simulink model "accumulator_thermal_model"  (R2021a)
settings: Solver=VariableStepAuto  StartTime=0.0  StopTime=Tend  RelTol=1e-7  AbsTol=1e-7
values from neighbouring files (symbols this model uses):
  AH = 13.5    [HT07_Simulink_Setup.m]    (also in Simulink_Setup.m = 17)
  cellInternalResis = .0018    (= 0.0018)    [Simulink_Setup.m]
  SOC0 = 1    [HT07_Simulink_Setup.m]    (also in Simulink_Setup.m)
  startTempC = 26    [HT07_Simulink_Setup.m]    (also in Simulink_Setup.m = 23.3)
  tabResis = 0.00010*nCell    (= 0.0126)    [HT07_Simulink_Setup.m]    (also in Simulink_Setup.m = 9e-05)
undefined symbols (not defined in the file or in its folder): DiscIntNeverNeededParam, emCurrent
libraries: fl_lib x42, nesl_utility x14, ee_lib x2
settings Model: OrderedModelArguments=off  Creator=elrii  LastModifiedBy=erc
settings SolverCC: AutoScaleAbsTol=off  AlgebraicLoopSolver=TrustRegion
settings DataIOCC: ReturnWorkspaceOutputsName=tp141c3138_a421_409b_bff7_0e00beb78378
settings DebuggingCC: SymbolicDimsDataTypeCodeGenerationDiagnostic=none  SFMachineParentedDataDiag=warning
settings SFSimCC: CustomCodeUndefinedFunction=UseInterfaceOnly
settings SimscapeCC: SimscapeLogType=all  SimscapeLogSimulationStatistics=on  SimscapeLogDataHistory=10000

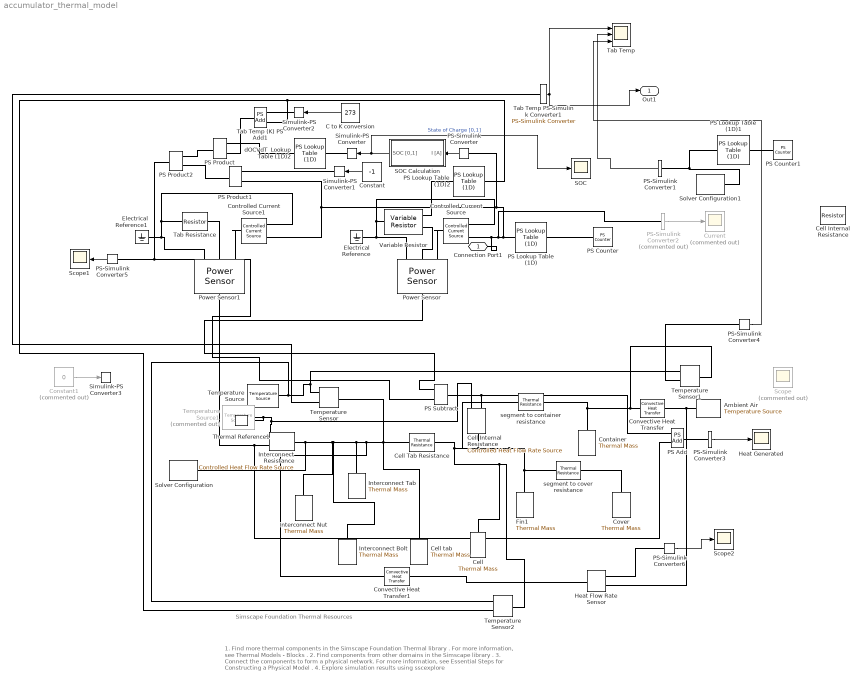
== system accumulator_thermal_model ==
  note: 1. Find more thermal components in the Simscape Foundation Thermal library .
      | For more information, see Thermal Models - Blocks .
      | 2. Find components from other domains in the Simscape library .
      | 3. Connect the components to form a physical network.
      | For more information, see Essential Steps for Constructing a Physical Model .
      | 4. Explore simulation results using sscexplore
  note: Simscape Foundation Thermal Resources
  " Fin1" : fl_lib/Thermal/Thermal Elements/Thermal Mass  mass=mFin kg  sp_heat=cAl J/kg/K  T_specify=on  T_priority=High  T=startTempC degC  T_nominal_specify=off  T_nominal_unit=K  T_nominal_value=1  Q_specify=off  Q_priority=None  Q=0 W  Q_nominal_specify=off  Q_nominal_unit=W  Q_nominal_value=1
  Ambient Air : fl_lib/Thermal/Thermal Sources/Temperature Source  temperature=startTempC degC
  C to K conversion : Constant  Value=273
  "Cell " : fl_lib/Thermal/Thermal Elements/Thermal Mass  mass=mCell kg  sp_heat=cCell J/kg/K  T_specify=on  T_priority=High  T=startTempC degC  T_nominal_specify=off  T_nominal_unit=K  T_nominal_value=1  Q_specify=off  Q_priority=None  Q=0 W  Q_nominal_specify=off  Q_nominal_unit=W  Q_nominal_value=1
  Cell Internal Resistance : fl_lib/Thermal/Thermal Sources/Controlled Heat Flow Rate Source
  "Cell Internal Resistance " : fl_lib/Electrical/Electrical Elements/Resistor  R=cellInternalResis Ohm  i_specify=off  i_priority=None  i=0 A  i_nominal_specify=off  i_nominal_unit=A  i_nominal_value=1  v_specify=off  v_priority=None  v=0 V  v_nominal_specify=off  v_nominal_unit=V  v_nominal_value=1  mask(Resistor){}
  Cell Tab Resistance : fl_lib/Thermal/Thermal Elements/Thermal Resistance  resistance=R_tc K/W  T_specify=off  T_priority=None  T=0 K  T_nominal_specify=off  T_nominal_unit=K  T_nominal_value=1  Q_specify=off  Q_priority=None  Q=0 W  Q_nominal_specify=off  Q_nominal_unit=W  Q_nominal_value=1
      settings: SourceProductBaseCode=SS
  Cell tab : fl_lib/Thermal/Thermal Elements/Thermal Mass  mass=cellTabThermalMass kg  sp_heat=cCu J/kg/K  T_specify=on  T_priority=High  T=startTempC degC  T_nominal_specify=off  T_nominal_unit=K  T_nominal_value=1  Q_specify=off  Q_priority=None  Q=0 W  Q_nominal_specify=off  Q_nominal_unit=W  Q_nominal_value=1
  Constant : Constant  Value=-1
  Constant1 : Constant  Commented=on  Value=0
  Container : fl_lib/Thermal/Thermal Elements/Thermal Mass  mass=mContainerAdj kg  sp_heat=cAl J/kg/K  T_specify=on  T_priority=High  T=startTempC degC  T_nominal_specify=off  T_nominal_unit=K  T_nominal_value=1  Q_specify=off  Q_priority=None  Q=0 W  Q_nominal_specify=off  Q_nominal_unit=W  Q_nominal_value=1
  Controlled Current Source : fl_lib/Electrical/Electrical Sources/Controlled Current Source
  Controlled Current Source1 : fl_lib/Electrical/Electrical Sources/Controlled Current Source
  Convective Heat Transfer : fl_lib/Thermal/Thermal Elements/Convective Heat Transfer  area=convectionArea m^2  heat_tr_coeff=10 W/(m^2 * K)  T_specify=off  T_priority=None  T=0 K  T_nominal_specify=off  T_nominal_unit=K  T_nominal_value=1  Q_specify=off  Q_priority=None  Q=0 W  Q_nominal_specify=off  Q_nominal_unit=W  Q_nominal_value=1
  Convective Heat Transfer1 : fl_lib/Thermal/Thermal Elements/Convective Heat Transfer  area=2.62e-4 m^2  heat_tr_coeff=.001 W/(m^2 * K)  T_specify=off  T_priority=None  T=0 K  T_nominal_specify=off  T_nominal_unit=K  T_nominal_value=1  Q_specify=off  Q_priority=None  Q=0 W  Q_nominal_specify=off  Q_nominal_unit=W  Q_nominal_value=1
  Cover : fl_lib/Thermal/Thermal Elements/Thermal Mass  mass=mCoverAdj kg  sp_heat=cAl J/kg/K  T_specify=on  T_priority=High  T=startTempC degC  T_nominal_specify=off  T_nominal_unit=K  T_nominal_value=1  Q_specify=off  Q_priority=None  Q=0 W  Q_nominal_specify=off  Q_nominal_unit=W  Q_nominal_value=1
  Current : Scope  Commented=on
  Electrical Reference : fl_lib/Electrical/Electrical Elements/Electrical Reference
  Electrical Reference1 : fl_lib/Electrical/Electrical Elements/Electrical Reference
  Heat Flow Rate Sensor : fl_lib/Thermal/Thermal Sensors/Heat Flow Rate Sensor
      settings: SourceProductBaseCode=SS
  Heat Generated : Scope
  Interconnect Bolt : fl_lib/Thermal/Thermal Elements/Thermal Mass  mass=mInterconnectBoltTotal kg  sp_heat=cSt J/kg/K  T_specify=on  T_priority=High  T=startTempC degC  T_nominal_specify=off  T_nominal_unit=K  T_nominal_value=1  Q_specify=off  Q_priority=None  Q=0 W  Q_nominal_specify=off  Q_nominal_unit=W  Q_nominal_value=1
  Interconnect Nut : fl_lib/Thermal/Thermal Elements/Thermal Mass  mass=mInterconnectNutTotal kg  sp_heat=cSt J/kg/K  T_specify=on  T_priority=High  T=startTempC degC  T_nominal_specify=off  T_nominal_unit=K  T_nominal_value=1  Q_specify=off  Q_priority=None  Q=0 W  Q_nominal_specify=off  Q_nominal_unit=W  Q_nominal_value=1
  Interconnect Resistance : fl_lib/Thermal/Thermal Sources/Controlled Heat Flow Rate Source
  Interconnect Tab : fl_lib/Thermal/Thermal Elements/Thermal Mass  mass=mInterconnect kg  sp_heat=cAl J/kg/K  T_specify=on  T_priority=High  T=startTempC degC  T_nominal_specify=off  T_nominal_unit=K  T_nominal_value=1  Q_specify=off  Q_priority=None  Q=0 W  Q_nominal_specify=off  Q_nominal_unit=W  Q_nominal_value=1
  PS Add : fl_lib/Physical Signals/Functions/PS Add
  PS Counter : fl_lib/Physical Signals/Sources/PS Counter  sample_time=1 s  init_val=1  reset_val=0  max_val=100000
      settings: SourceProductBaseCode=SS  InternalSimscapePortConfiguration="{\"Bottom\":[],\"Left\":[],\"Right\":[{\"id\":\"Y\",\"label\":\"Y\",\"type\":\"output\"}],\"Top\":[]}"
  PS Counter1 : fl_lib/Physical Signals/Sources/PS Counter  sample_time=1 s  init_val=1  reset_val=0  max_val=100000
      settings: SourceProductBaseCode=SS  InternalSimscapePortConfiguration="{\"Bottom\":[],\"Left\":[],\"Right\":[{\"id\":\"Y\",\"label\":\"Y\",\"type\":\"output\"}],\"Top\":[]}"
  PS Lookup Table (1D) : fl_lib/Physical Signals/Lookup Tables/PS Lookup Table (1D)  x=emTime  f=-emCurrent A  interp_method=simscape.enum.interpolation.linear  extrap_method=simscape.enum.extrapolation.nearest
      settings: SourceProductBaseCode=SS
  PS Lookup Table (1D)1 : fl_lib/Physical Signals/Lookup Tables/PS Lookup Table (1D)  x=time  f=tempInterp  interp_method=simscape.enum.interpolation.linear  extrap_method=simscape.enum.extrapolation.nearest
      settings: SourceProductBaseCode=SS
  PS Lookup Table (1D)2 : fl_lib/Physical Signals/Lookup Tables/PS Lookup Table (1D)  x=tempVec K  f=IRVec Ohm  interp_method=simscape.enum.interpolation.linear  extrap_method=simscape.enum.extrapolation.linear
      settings: SourceProductBaseCode=SS
  PS Product : fl_lib/Physical Signals/Functions/PS Product
  PS Product1 : fl_lib/Physical Signals/Functions/PS Product
  PS Product2 : fl_lib/Physical Signals/Functions/PS Product
  PS Subtract : fl_lib/Physical Signals/Functions/PS Subtract
  PS-Simulink Converter{,1,3..6} (6 alike) : nesl_utility/PS-Simulink Converter  PhysicalDomain=network_engine_domain  SubClassName=ps_output  LeftPortType=input  RightPortType=output  PseudoPeriodic=off  Frequencies=[]  Unit=inherit  AffineConversion=off
      settings: SourceProductBaseCode=PW,SS
  PS-Simulink Converter2 : nesl_utility/PS-Simulink Converter  Commented=on  PhysicalDomain=network_engine_domain  SubClassName=ps_output  LeftPortType=input  RightPortType=output  PseudoPeriodic=off  Frequencies=[]  Unit=inherit  AffineConversion=off
      settings: SourceProductBaseCode=PW,SS
  Power Sensor : ee_lib/Sensors & Transducers/Power Sensor  measurement_type=1  averaging_period=1e-4 s
      settings: SourceProductBaseCode=PS
  Power Sensor1 : ee_lib/Sensors & Transducers/Power Sensor  measurement_type=1  averaging_period=1e-4 s
      settings: SourceProductBaseCode=PS
  SOC : Scope
  SOC Calculation : Subsystem
  Scope : Scope  Commented=on
  Scope1 : Scope
  Scope2 : Scope
  Simulink-PS Converter : nesl_utility/Simulink-PS Converter  PhysicalDomain=network_engine_domain  SubClassName=ps_input  LeftPortType=input  RightPortType=output  PseudoPeriodic=off  Frequencies=[]  NoiseDistribution=none  NoiseParameters=[]  Unit=1  AffineConversion=off  FilteringAndDerivatives=provide  SimscapeFilterOrder=1  InputFilterTimeConstant=0.001  UdotUserProvided=0
      settings: SourceProductBaseCode=PW,SS
  Simulink-PS Converter1 : nesl_utility/Simulink-PS Converter  PhysicalDomain=network_engine_domain  SubClassName=ps_input  LeftPortType=input  RightPortType=output  PseudoPeriodic=off  Frequencies=[]  NoiseDistribution=none  NoiseParameters=[]  Unit=1  AffineConversion=off  FilteringAndDerivatives=provide  SimscapeFilterOrder=1  InputFilterTimeConstant=0.001  UdotUserProvided=0
      settings: SourceProductBaseCode=PW,SS
  Simulink-PS Converter2 : nesl_utility/Simulink-PS Converter  PhysicalDomain=network_engine_domain  SubClassName=ps_input  LeftPortType=input  RightPortType=output  PseudoPeriodic=off  Frequencies=[]  NoiseDistribution=none  NoiseParameters=[]  Unit=K  AffineConversion=off  FilteringAndDerivatives=provide  SimscapeFilterOrder=1  InputFilterTimeConstant=0.001  UdotUserProvided=0
      settings: SourceProductBaseCode=PW,SS
  Simulink-PS Converter3 : nesl_utility/Simulink-PS Converter  PhysicalDomain=network_engine_domain  SubClassName=ps_input  LeftPortType=input  RightPortType=output  PseudoPeriodic=off  Frequencies=[]  NoiseDistribution=none  NoiseParameters=[]  Unit=W  AffineConversion=off  FilteringAndDerivatives=provide  SimscapeFilterOrder=1  InputFilterTimeConstant=0.001  UdotUserProvided=0
      settings: SourceProductBaseCode=PW,SS
  Solver Configuration : nesl_utility/Solver Configuration  PhysicalDomain=network_engine_domain  SubClassName=solver  LeftPortType=input  RightPortType=generic  Tones=[]  Harmonics=[]  SimulateNoise=off  Profile=off  UseLocalSampling=off  EnableSwitchedLinearOptims=on  FrequencyDomain=off  UseCCode=off  RelTol=0.001  AbsTol=1e-06  MinStep=1e-09  ToWorkspace=off  RevertToSquareIcSolve=off  NumHomotopyIterations=100  PhasorMode=off  PhasorModeNumHarmonics=1  DoDC=off  ResidualTolerance=1e-012  UseLocalSolver=off  LocalSolverChoice=NE_BACKWARD_EULER_ADVANCER  LocalSolverSampleTime=0.001  DoFixedCost=off  MaxNonlinIter=3  MaxModeIter=2  ComputeImpulses=off  ImpulseIterations=2  LinearAlgebra=auto  EquationFormulation=NE_TIME_EF  DelaysMemoryBudget=1024  AutomaticFiltering=on  FilteringTimeConstant=0.001  PartitionStorageMethod=AS_NEEDED  PartitionMemoryBudget=1024  PartitionMethod=ROBUST
      settings: SourceProductBaseCode=PW,SS
  Solver Configuration1 : nesl_utility/Solver Configuration  PhysicalDomain=network_engine_domain  SubClassName=solver  LeftPortType=input  RightPortType=generic  Tones=[]  Harmonics=[]  SimulateNoise=off  Profile=off  UseLocalSampling=off  EnableSwitchedLinearOptims=on  FrequencyDomain=off  UseCCode=off  RelTol=0.001  AbsTol=1e-06  MinStep=1e-09  ToWorkspace=off  RevertToSquareIcSolve=off  NumHomotopyIterations=100  PhasorMode=off  PhasorModeNumHarmonics=1  DoDC=off  ResidualTolerance=1e-09  UseLocalSolver=off  LocalSolverChoice=NE_BACKWARD_EULER_ADVANCER  LocalSolverSampleTime=0.001  DoFixedCost=off  MaxNonlinIter=3  MaxModeIter=2  ComputeImpulses=off  ImpulseIterations=2  LinearAlgebra=auto  EquationFormulation=NE_TIME_EF  DelaysMemoryBudget=1024  AutomaticFiltering=on  FilteringTimeConstant=0.001  PartitionStorageMethod=AS_NEEDED  PartitionMemoryBudget=1024  PartitionMethod=ROBUST
      settings: SourceProductBaseCode=PW,SS
  Tab Resistance : fl_lib/Electrical/Electrical Elements/Resistor  R=tabResis Ohm  i_specify=off  i_priority=None  i=0 A  i_nominal_specify=off  i_nominal_unit=A  i_nominal_value=1  v_specify=off  v_priority=None  v=0 V  v_nominal_specify=off  v_nominal_unit=V  v_nominal_value=1  mask(Resistor){}
  Tab Temp : Scope  NumInputPorts=3
  Tab Temp (K) PS Add1 : fl_lib/Physical Signals/Functions/PS Add
  Tab Temp PS-Simulink Converter1 : nesl_utility/PS-Simulink Converter  PhysicalDomain=network_engine_domain  SubClassName=ps_output  LeftPortType=input  RightPortType=output  PseudoPeriodic=off  Frequencies=[]  Unit=inherit  AffineConversion=off
      settings: SourceProductBaseCode=PW,SS
  Temperature Sensor : fl_lib/Thermal/Thermal Sensors/Temperature Sensor
  Temperature Sensor1 : fl_lib/Thermal/Thermal Sensors/Temperature Sensor
  Temperature Sensor2 : fl_lib/Thermal/Thermal Sensors/Temperature Sensor
  Temperature Source : fl_lib/Thermal/Thermal Sources/Temperature Source  temperature=0 degC
  Temperature Source1 : fl_lib/Thermal/Thermal Sources/Temperature Source  Commented=on  temperature=0 degC
  Thermal Reference1 : fl_lib/Thermal/Thermal Elements/Thermal Reference
  Variable Resistor : fl_lib/Electrical/Electrical Elements/Variable Resistor  Rmin=0 Ohm  i_specify=off  i_priority=None  i=0 A  i_nominal_specify=off  i_nominal_unit=A  i_nominal_value=1  v_specify=off  v_priority=None  v=0 V  v_nominal_specify=off  v_nominal_unit=V  v_nominal_value=1
  dOCVdT  Lookup Table (1D)2 : fl_lib/Physical Signals/Lookup Tables/PS Lookup Table (1D)  x=SOC  f=dOCVdT V/K  interp_method=simscape.enum.interpolation.linear  extrap_method=simscape.enum.extrapolation.linear
      settings: SourceProductBaseCode=SS
  segment to container resistance : fl_lib/Thermal/Thermal Elements/Thermal Resistance  resistance=R_cb K/W  T_specify=off  T_priority=None  T=0 K  T_nominal_specify=off  T_nominal_unit=K  T_nominal_value=1  Q_specify=off  Q_priority=None  Q=0 W  Q_nominal_specify=off  Q_nominal_unit=W  Q_nominal_value=1
      settings: SourceProductBaseCode=SS
  segment to cover resistance : fl_lib/Thermal/Thermal Elements/Thermal Resistance  resistance=R_cb K/W  T_specify=off  T_priority=None  T=0 K  T_nominal_specify=off  T_nominal_unit=K  T_nominal_value=1  Q_specify=off  Q_priority=None  Q=0 W  Q_nominal_specify=off  Q_nominal_unit=W  Q_nominal_value=1
      settings: SourceProductBaseCode=SS
  Connection Port1 : PMIOPort  Side=Left
  Out1 : Outport
  wires:
  PS-Simulink Converter2/1 -> Current/1
  PS-Simulink Converter3/1 -> Heat Generated/1
  Tab Temp PS-Simulink Converter1/1 -> Out1/1, Tab Temp/1
  PS-Simulink Converter1/1 -> Tab Temp/2
  PS-Simulink Converter/1 -> SOC Calculation/1(I [A])
  SOC Calculation/1(SOC [0,1]) -> SOC/1, Simulink-PS Converter/1  "State of Charge [0,1]"
  Constant/1 -> Simulink-PS Converter1/1
  C to K conversion/1 -> Simulink-PS Converter2/1
  PS-Simulink Converter5/1 -> Scope1/1
  Constant1/1 -> Simulink-PS Converter3/1
  PS-Simulink Converter4/1 -> Tab Temp/3
  PS-Simulink Converter6/1 -> Scope2/1
  connections:
  segment to cover resistance/LConn1 -- " Fin1"/LConn1 -- segment to container resistance/LConn1 -- Cell Internal Resistance/LConn1 -- Cell Tab Resistance/RConn1 -- Temperature Sensor2/LConn1 -- "Cell "/LConn1
  Interconnect Resistance/LConn1 -- Convective Heat Transfer1/LConn1 -- Cell tab/LConn1 -- Cell Tab Resistance/LConn1 -- Temperature Sensor/LConn1 -- Interconnect Tab/LConn1 -- Interconnect Bolt/LConn1 -- Interconnect Nut/LConn1 -- Solver Configuration/RConn1
  Controlled Current Source/LConn1 -- Power Sensor/LConn1
  Power Sensor/LConn2 -- Variable Resistor/LConn2
  Power Sensor/LConn3 -- Electrical Reference/LConn1 -- Variable Resistor/RConn1 -- Controlled Current Source/RConn2
  Tab Resistance/RConn1 -- Controlled Current Source1/RConn2 -- Power Sensor1/LConn3 -- Electrical Reference1/LConn1
  Tab Resistance/LConn1 -- Power Sensor1/LConn2
  Controlled Current Source1/LConn1 -- Power Sensor1/LConn1
  Power Sensor1/RConn1 -- PS Add/LConn2 -- Interconnect Resistance/RConn1
  Cell Internal Resistance/RConn2 -- Thermal Reference1/LConn1 -- Temperature Source1/LConn1 -- Interconnect Resistance/RConn2
  segment to container resistance/RConn1 -- Temperature Sensor1/LConn1 -- Convective Heat Transfer/LConn1 -- Container/LConn1
  Controlled Current Source/RConn1 -- Connection Port1/RConn1 -- PS-Simulink Converter2/LConn1 -- PS-Simulink Converter/LConn1 -- PS Product1/LConn2 -- Controlled Current Source1/RConn1 -- PS Lookup Table (1D)/RConn1
  PS Counter/RConn1 -- PS Lookup Table (1D)/LConn1
  Temperature Source/LConn1 -- Temperature Sensor2/RConn1 -- Temperature Sensor1/RConn1 -- Temperature Sensor/RConn1
  PS Add/RConn1 -- PS-Simulink Converter3/LConn1
  PS Lookup Table (1D)1/RConn1 -- Solver Configuration1/RConn1 -- PS-Simulink Converter1/LConn1
  PS Lookup Table (1D)1/LConn1 -- PS Counter1/RConn1
  Tab Temp PS-Simulink Converter1/LConn1 -- Temperature Sensor/RConn2
  Simulink-PS Converter/RConn1 -- dOCVdT  Lookup Table (1D)2/LConn1
  dOCVdT  Lookup Table (1D)2/RConn1 -- PS Product/LConn1
  PS Product1/LConn1 -- Simulink-PS Converter1/RConn1
  PS Product2/LConn1 -- PS Product/RConn1
  PS Product1/RConn1 -- PS Product2/LConn2
  PS Subtract/LConn1 -- Power Sensor/RConn1
  PS Add/LConn1 -- PS Subtract/RConn1 -- Cell Internal Resistance/RConn1
  Tab Temp (K) PS Add1/LConn1 -- Simulink-PS Converter2/RConn1
  PS Product/LConn2 -- Tab Temp (K) PS Add1/RConn1
  PS-Simulink Converter4/LConn1 -- Temperature Sensor1/RConn2
  Convective Heat Transfer/RConn1 -- Heat Flow Rate Sensor/RConn2 -- Ambient Air/LConn1
  PS-Simulink Converter5/LConn1 -- PS Subtract/LConn2 -- PS Product2/RConn1
  PS Lookup Table (1D)2/RConn1 -- Variable Resistor/LConn1
  Temperature Sensor2/RConn2 -- Tab Temp (K) PS Add1/LConn2 -- PS Lookup Table (1D)2/LConn1
  segment to cover resistance/RConn1 -- Cover/LConn1
  Convective Heat Transfer1/RConn1 -- Heat Flow Rate Sensor/LConn1
  Heat Flow Rate Sensor/RConn1 -- PS-Simulink Converter6/LConn1

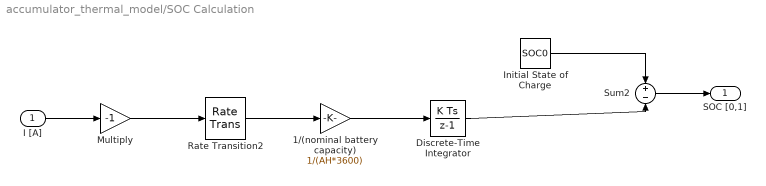
== system accumulator_thermal_model/SOC Calculation ==
  I [A] : Inport
  1/(nominal battery capacity) : Gain  Gain=1/(AH*3600)
  Discrete-Time Integrator : DiscreteIntegrator  SampleTime=-1  ICPrevOutput=DiscIntNeverNeededParam  ICPrevScaledInput=DiscIntNeverNeededParam
  Initial State of Charge : Constant  Value=SOC0
  Multiply : Gain  Gain=-1
  Rate Transition2 : RateTransition
  Sum2 : Sum  Inputs=+-
  SOC [0,1] : Outport  VectorParamsAs1DForOutWhenUnconnected=off
  wires:
  Rate Transition2/1 -> 1/(nominal battery capacity)/1
  1/(nominal battery capacity)/1 -> Discrete-Time Integrator/1
  Initial State of Charge/1 -> Sum2/1
  Discrete-Time Integrator/1 -> Sum2/2
  Sum2/1 -> SOC [0,1]/1
  I [A]/1 -> Multiply/1
  Multiply/1 -> Rate Transition2/1
